simulink model "PID_lead_controllers_linmod2"  (R2023b)
settings: Solver=ode8  StartTime=0.0  StopTime=20  FixedStep=0.001  RelTol=1e-3
values from neighbouring files (symbols this model uses):
  K = p/z    [lead_vs_leadlag.m]    (also in setup_lead_controller.m)
  p = bodeoptions    [PID_lead_linmod.m]    (also in lead_vs_leadlag.m = 1/(alpha*T); setup_lead_controller.m = 1/(alpha*T))
  z = 1/T    [lead_vs_leadlag.m]    (also in setup_lead_controller.m)
settings Model: Creator=suvo  LastModifiedBy=suvo
settings SolverCC: AlgebraicLoopSolver=TrustRegion
settings DataIOCC: ReturnWorkspaceOutputs=off
settings DebuggingCC: UnconnectedInputMsg=warning  UnconnectedOutputMsg=warning  UnconnectedLineMsg=warning
settings ModelReferenceCC: EnableRefExpFcnMdlSchedulingChecks=on

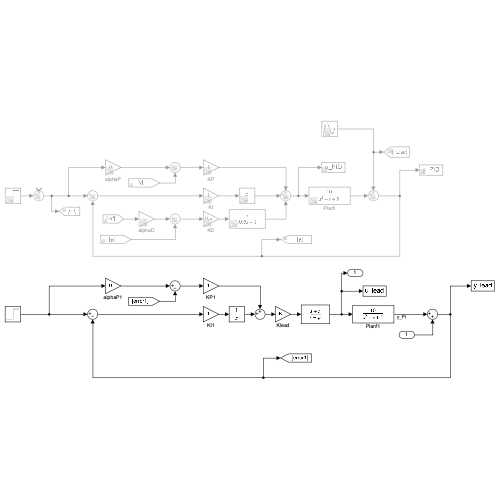
[thumbnail: Simulink's stored preview of the top-level diagram]
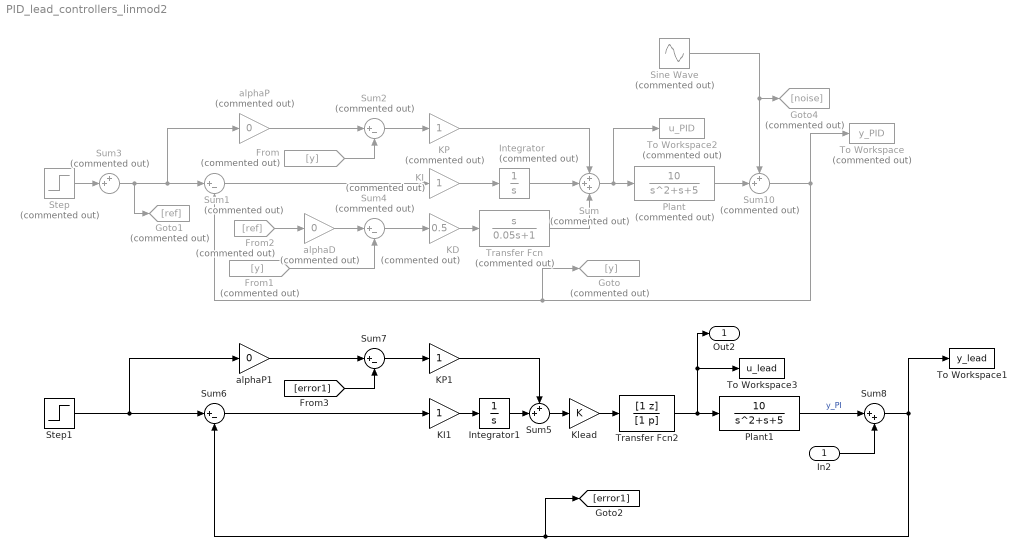
== system PID_lead_controllers_linmod2 ==
  In2 : Inport
  From : From  Commented=on  GotoTag=y
  From1 : From  Commented=on  GotoTag=y
  From2 : From  Commented=on  GotoTag=ref
  Goto : Goto  Commented=on  GotoTag=y
  Goto1 : Goto  Commented=on  GotoTag=ref
  Goto4 : Goto  Commented=on  GotoTag=noise
  Integrator : Integrator  Commented=on
  Integrator1 : Integrator
  KD : Gain  Commented=on  Gain=0.5
  KI : Gain  Commented=on
  KI1 : Gain
  KP : Gain  Commented=on
  KP1 : Gain
  Klead : Gain  Gain=K
  Plant : TransferFcn  Commented=on  Numerator=10  Denominator=[1 1 5]
  Plant1 : TransferFcn  Numerator=10  Denominator=[1 1 5]
  Sine Wave : Sin  Commented=on  Amplitude=0.01  Frequency=20  SampleTime=0
  Step : Step  Commented=on  SampleTime=0
  Step1 : Step  SampleTime=0
  Sum : Sum  Commented=on  Inputs=+++
  Sum1 : Sum  Commented=on  Inputs=|+-
  Sum10 : Sum  Commented=on  Inputs=++|
  Sum2 : Sum  Commented=on  Inputs=|+-
  Sum3 : Sum  Commented=on  Inputs=++|
  Sum4 : Sum  Commented=on  Inputs=|+-
  Sum5 : Sum  Inputs=++|
  Sum6 : Sum  Inputs=|+-
  Sum7 : Sum  Inputs=|+-
  Sum8 : Sum  Inputs=|++
  To Workspace : ToWorkspace  Commented=on  VariableName=y_PID  SaveFormat=Timeseries  SampleTime=-1
  To Workspace1 : ToWorkspace  VariableName=y_lead  SaveFormat=Timeseries  SampleTime=-1
  To Workspace2 : ToWorkspace  Commented=on  VariableName=u_PID  SaveFormat=Timeseries  SampleTime=-1
  To Workspace3 : ToWorkspace  VariableName=u_lead  SaveFormat=Timeseries  SampleTime=-1
  Transfer Fcn : TransferFcn  Commented=on  Numerator=[1 0]  Denominator=[0.05 1]
  Transfer Fcn2 : TransferFcn  Numerator=[1 z]  Denominator=[1 p]
  alphaD : Gain  Commented=on  Gain=0
  alphaP : Gain  Commented=on  Gain=0
  alphaP1 : Gain  Gain=0
  Out2 : Outport
  wires:
  KI/1 -> Integrator/1
  Sum1/1 -> KI/1
  Sum3/1 -> alphaP/1, Sum1/1, Goto1/1
  Sum2/1 -> KP/1
  KP/1 -> Sum/1
  Integrator/1 -> Sum/2
  Sum/1 -> To Workspace2/1, Plant/1
  Step/1 -> Sum3/2
  From/1 -> Sum2/2
  KD/1 -> Transfer Fcn/1
  Transfer Fcn/1 -> Sum/3
  Sum4/1 -> KD/1
  From1/1 -> Sum4/2
  From2/1 -> alphaD/1
  alphaP/1 -> Sum2/1
  Sum6/1 -> KI1/1
  KP1/1 -> Sum5/1
  KI1/1 -> Integrator1/1
  Sum7/1 -> KP1/1
  [error1] -> Sum7/2
  Integrator1/1 -> Sum5/2
  Step1/1 -> alphaP1/1, Sum6/1
  Sum5/1 -> Klead/1
  alphaP1/1 -> Sum7/1
  Plant/1 -> Sum10/2
  Sum10/1 -> To Workspace/1, Goto/1, Sum1/2
  Sine Wave/1 -> Sum10/1, Goto4/1
  Transfer Fcn2/1 -> Out2/1, To Workspace3/1, Plant1/1
  alphaD/1 -> Sum4/1
  Klead/1 -> Transfer Fcn2/1
  Plant1/1 -> Sum8/1  "y_PI"
  Sum8/1 -> [error1], Sum6/2, To Workspace1/1
  In2/1 -> Sum8/2
